simulink model "Carol_Arduino_observador_2021"  (R2021a)
settings: Solver=ode4  StartTime=0.0  StopTime=inf  FixedStep=0.001  RelTol=1e-3  EnableMultiTasking=on
libraries: arduinolib x2
settings Model: SILPILModeSetting=veronly  ExtModeTrigDuration=2  Creator=lcauf  LastModifiedBy=lcauf
settings OptimizationCC: EnhancedBackFolding=on  PassReuseOutputArgsAs=Individual arguments  ZeroExternalMemoryAtStartup=off  ZeroInternalMemoryAtStartup=off  MaxStackSize=64  OptimizeBlockOrder=speed  DifferentSizesBufferReuse=on  OptimizationCustomize=off  EfficientTunableParamExpr=on
settings DebuggingCC: ParameterTunabilityLossMsg=error
settings HardwareCC: ProdBitPerPointer=32  ProdBitPerSizeT=32  ProdBitPerPtrDiffT=32  ProdLargestAtomicInteger=Long  ProdLargestAtomicFloat=Double  ProdWordSize=32  ProdHWDeviceType=ARM Compatible->ARM Cortex  UseEmbeddedCoderFeatures=off
settings SFSimCC: MATLABDynamicMemAlloc=off
settings RTWCC: SystemTargetFile=ert.tlc  HardwareBoard=Arduino Due  TemplateMakefile=ert_default_tmf  Toolchain=Arduino ARM  BuildConfiguration=Faster Runs
settings CodeAppCC: ForceParamTrailComments=on  IgnoreCustomStorageClasses=off  OperatorAnnotations=on  SimulinkDataObjDesc=on  SFDataObjDesc=on  InsertBlockDesc=on
settings ERTTargetCC: SupportContinuousTime=on  SupportNonInlinedSFcns=on  SupportVariableSizeSignals=on  ExtModeTransport=3  ExtModeStaticAlloc=on  ExtModeStaticAllocSize=24576  ExtModeMexFile=ext_xcp  ExtModeIntrfLevel=Level2 - Open

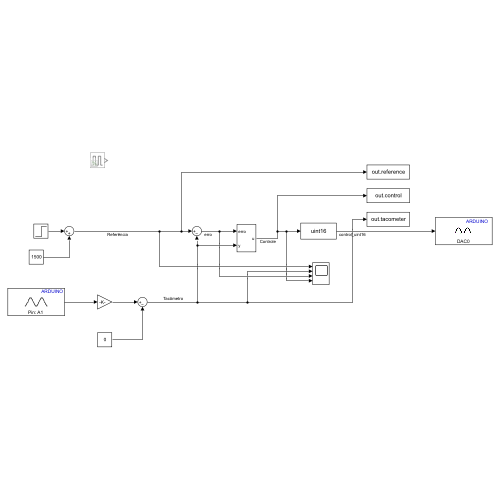
[thumbnail: Simulink's stored preview of the top-level diagram]
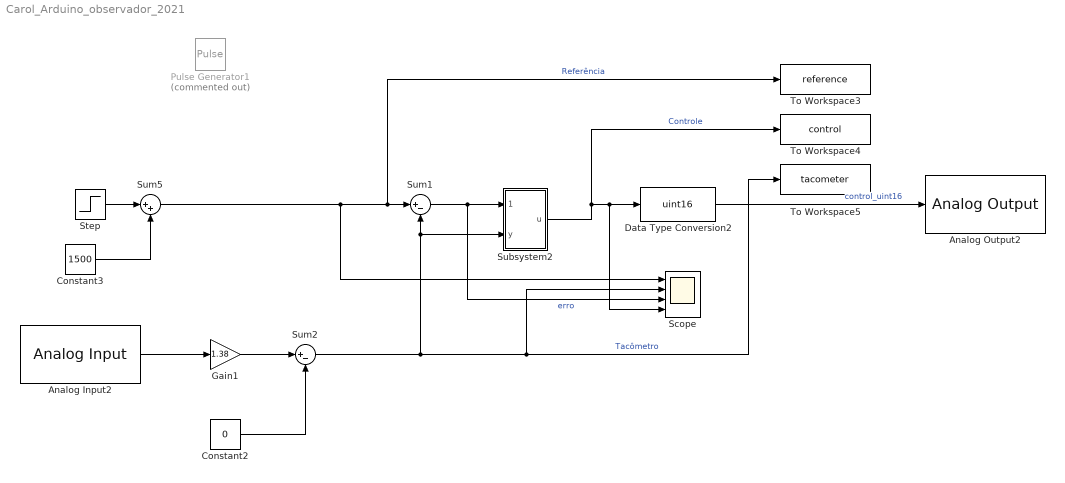
== system Carol_Arduino_observador_2021 ==
  Analog Input2 : arduinolib/Analog Input  pinNumber=1  ReadResultsOnly=off  ConversionTriggerSource=Software  ExternalTriggerType=uint32( 0 )  OutputDataType=uint16  EnableConversionCompleteNotify=off  EnableOuputStatus=off  SampleTime=-1  blockPlatform=arduino
  Analog Output2 : arduinolib/Analog Output  DACpin=DAC0  blockPlatform=arduino
      settings: SourceProductBaseCode=ARDUINO
  Constant2 : Constant  Value=0
  Constant3 : Constant  Value=1500
  Data Type Conversion2 : DataTypeConversion  OutDataTypeStr=uint16
  Gain1 : Gain  Gain=1.38
  Pulse Generator1 : DiscretePulseGenerator  Commented=on  PulseType=Time based  Amplitude=2000  PulseWidth=50
  Scope : Scope  NumInputPorts=4
  Step : Step  After=2000  SampleTime=0
  Subsystem2 : Subsystem
  Sum1 : Sum  Inputs=|+-
  Sum2 : Sum  Inputs=|+-
  Sum5 : Sum  Inputs=|++
  To Workspace3 : ToWorkspace  VariableName=reference  SaveFormat=Structure With Time  SampleTime=-1
  To Workspace4 : ToWorkspace  VariableName=control  SaveFormat=Structure With Time  SampleTime=-1
  To Workspace5 : ToWorkspace  VariableName=tacometer  SaveFormat=Structure With Time  SampleTime=-1
  wires:
  Constant2/1 -> Sum2/2
  Sum1/1 -> Scope/3, Subsystem2/1(erro)  "erro"
  Analog Input2/1 -> Gain1/1
  Data Type Conversion2/1 -> Analog Output2/1  "control_uint16"
  Sum5/1 -> Scope/1, To Workspace3/1, Sum1/1  "Referência"
  Subsystem2/1(u) -> To Workspace4/1, Scope/4, Data Type Conversion2/1  "Controle"
  Constant3/1 -> Sum5/2
  Sum2/1 -> Scope/2, To Workspace5/1, Sum1/2, Subsystem2/2(y)  "Tacômetro"
  Gain1/1 -> Sum2/1
  Step/1 -> Sum5/1

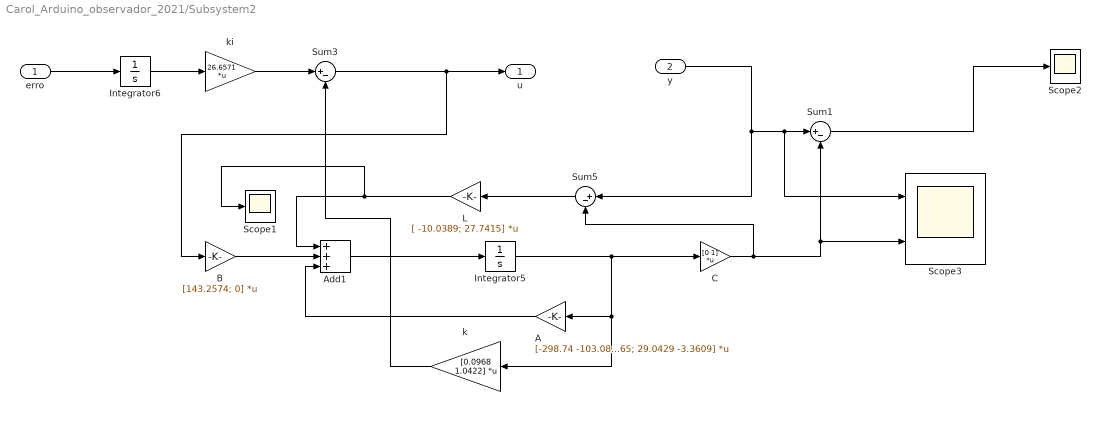
== system Carol_Arduino_observador_2021/Subsystem2 ==
  erro : Inport
  y : Inport  Port=2
  A : Gain  Gain=[-298.74 -103.0865; 29.0429 -3.3609]  Multiplication=Matrix(K*u)
  Add1 : Sum  Inputs=+++
  B : Gain  Gain=[143.2574; 0]  Multiplication=Matrix(K*u)
  C : Gain  Gain=[0 1]  Multiplication=Matrix(K*u)
  Integrator5 : Integrator  InitialCondition=-2
  Integrator6 : Integrator
  L : Gain  Gain=[ -10.0389; 27.7415]  Multiplication=Matrix(K*u)
  Scope1 : Scope
  Scope2 : Scope
  Scope3 : Scope  NumInputPorts=2
  Sum1 : Sum  Inputs=|+-
  Sum3 : Sum  Inputs=|+-
  Sum5 : Sum  Inputs=|+-
  k : Gain  Gain=[0.0968 1.0422]  Multiplication=Matrix(K*u)
  ki : Gain  Gain=26.6571  Multiplication=Matrix(K*u)
  u : Outport
  wires:
  k/1 -> Sum3/2
  Integrator6/1 -> ki/1
  y/1 -> Sum5/1, Scope3/1, Sum1/1
  erro/1 -> Integrator6/1
  Integrator5/1 -> C/1, k/1, A/1
  Sum5/1 -> L/1
  B/1 -> Add1/2
  ki/1 -> Sum3/1
  Add1/1 -> Integrator5/1
  L/1 -> Add1/1, Scope1/1
  C/1 -> Sum1/2, Scope3/2, Sum5/2
  A/1 -> Add1/3
  Sum1/1 -> Scope2/1
  Sum3/1 -> u/1, B/1
